simulink model "Turntable_sweep_2017"  (R2017b)
settings: Solver=ode4  StartTime=0.0  StopTime=10  FixedStep=0.0001  RelTol=1e-3
values from neighbouring files (symbols this model uses):
  b1 = 1 / taum    (= 1.01536120225)    [ESO.m]    (also in filter.m = 256.180350967; para_test.m)
  b2 = 1 / taue    (= 256.180350967)    [ESO.m]    (also in filter.m = 1.01536120225; para_test.m)
  beta1 = para.beta2    [ESO.m]    (also in filter.m = 221.733804685; myfun.m = x(6); para_test.m = 0.9528 * wq - b1 - b2)
  beta2 = para.beta3    [ESO.m]    (also in filter.m = 310055.997275; myfun.m = x(7); para_test.m = 1.4539 * wq * wq - b2 * beta1 - b1 * beta1 - b1 * b2)
  beta3 = para.beta4    [ESO.m]    (also in filter.m = 14508719.8625; myfun.m = x(8); para_test.m = 0.7426 * wq ^ 3 - b2 * beta2 - b1 * beta2 - b1 * b2 * beta1)
  beta4 = 0.2756 * wq ^ 4    (= 17593758835.7)    [filter.m]    (also in para_test.m = 0.2756 * wq ^ 4)
  fre = fre_array(i)    [sweep.m]
  gain = b0    (= 23249.4996924)    [para_test.m]
  J = 1.076    [sweep.m]
  Kps = 1.077250780790937e+02    (= 107.725078079)    [sweep.m]
  Kt = 24.812626200641272    (= 24.8126262006)    [sweep.m]
  Kv = 0.12    [sweep.m]
  L = 0.733240176511722    (= 0.733240176512)    [sweep.m]
  r = 80.116666666666666667    (= 80.1166666667)    [sweep.m]
  t_off = 10    [sweep.m]
  Type = 1    [sweep.m]
settings Model: Creator=Vera  LastModifiedBy=57531
settings SolverCC: AlgebraicLoopSolver=LineSearch
settings OptimizationCC: LifeSpan=inf
settings DebuggingCC: SFExecutionAtInitializationDiag=none
settings CodeAppCC: StateflowObjectComments=on

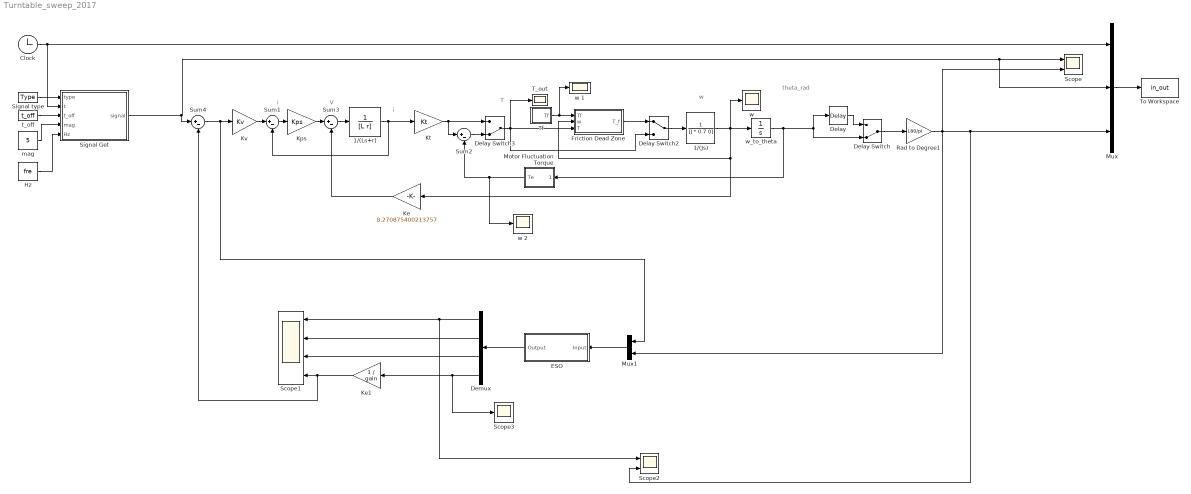
== system Turntable_sweep_2017 ==
  note: i
  note: w
  note: V
  note: i
  note: T
  note: theta_rad
  " Delay Switch" : ManualSwitch  CurrentSetting=0
  " Delay Switch2" : ManualSwitch
  " Delay Switch3" : ManualSwitch  CurrentSetting=0
  1/(Js) : TransferFcn  Denominator=[J * 0.7 0]
  1/(Ls+r) : TransferFcn  Denominator=[L r]
  Clock : Clock
  Delay : TransportDelay  DelayTime=0.003763900000000
  Demux : Demux
  ESO : Subsystem  mask{beta0=beta1, beta1=beta2, beta2=beta3, beta3=beta4, alpha1=0.5, alpha2=0.25, alpha3=0.125, delta1=0.01, delta2=0.01, delta3=0.01, h=0.0002, b0=gain}
  Friction Dead Zone : MATLAB Function  TreatAsAtomicUnit=on
  Hz : Constant  Value=fre
  Ke : Gain  Gain=8.270875400213757
  Ke1 : Gain  Gain=1 / gain
  Kps : Gain  Gain=Kps
  Kt : Gain  Gain=Kt
  Kv : Gain  Gain=Kv
  Motor Fluctuation Torque : Subsystem
  Mux : Mux  Inputs=3
  Mux1 : Mux  Inputs=2
  Rad to Degree1 : Gain  Gain=180/pi
  Scope : Scope  NumInputPorts=2
  Scope1 : Scope  NumInputPorts=4
  Scope2 : Scope  NumInputPorts=2
  Scope3 : Scope
  Signal Get : MATLAB Function  TreatAsAtomicUnit=on
  Signal type : Constant  Value=Type
  Sum{1..4} (4 alike) : Sum  Inputs=|+-
  T_out : Scope
  Tf : Subsystem
  To Workspace : ToWorkspace  VariableName=in_out  SampleTime=-1
  mag : Constant  Value=5
  t_off : Constant  Value=t_off
  "w " : Scope
  w 1 : Scope
  w 2 : Scope
  w_to_theta : Integrator
  wires:
  t_off/1 -> Signal Get/3(t_off)
  Clock/1 -> Mux/1, Signal Get/2(t)
  mag/1 -> Signal Get/4(mag)
  Hz/1 -> Signal Get/5(Hz)
  Kv/1 -> Sum1/1
  Motor Fluctuation Torque/1(Te) -> w 2/1, Sum2/2
  Tf/1(Tf) -> w 1/1, Friction Dead Zone/1(Tf)
  1/(Ls+r)/1 -> Sum1/2, Kt/1
  Sum3/1 -> 1/(Ls+r)/1
  Delay/1 -> " Delay Switch"/1
  w_to_theta/1 -> Delay/1, " Delay Switch"/2, Motor Fluctuation Torque/1(theta)
  " Delay Switch"/1 -> Rad to Degree1/1
  1/(Js)/1 -> "w "/1, w_to_theta/1, Friction Dead Zone/2(w), Ke/1
  " Delay Switch2"/1 -> 1/(Js)/1
  " Delay Switch3"/1 -> T_out/1, " Delay Switch2"/2, Friction Dead Zone/3(T)
  Ke/1 -> Sum3/2
  Sum2/1 -> " Delay Switch3"/2
  Sum1/1 -> Kps/1
  Kt/1 -> " Delay Switch3"/1, Sum2/1
  Kps/1 -> Sum3/1
  Mux/1 -> To Workspace/1
  Signal type/1 -> Signal Get/1(type)
  Rad to Degree1/1 -> Mux1/2, Scope2/2, Mux/3, Scope/2
  Demux/1 -> Scope2/1, Scope1/1
  Demux/2 -> Scope1/2
  Demux/3 -> Scope1/3
  Demux/4 -> Scope3/1, Ke1/1
  Friction Dead Zone/1(T_f) -> " Delay Switch2"/1
  Mux1/1 -> ESO/1(Input)
  ESO/1(Output) -> Demux/1
  Signal Get/1(signal) -> Sum4/1, Mux/2, Scope/1
  Ke1/1 -> Sum4/2, Scope1/4
  Sum4/1 -> Mux1/1, Kv/1

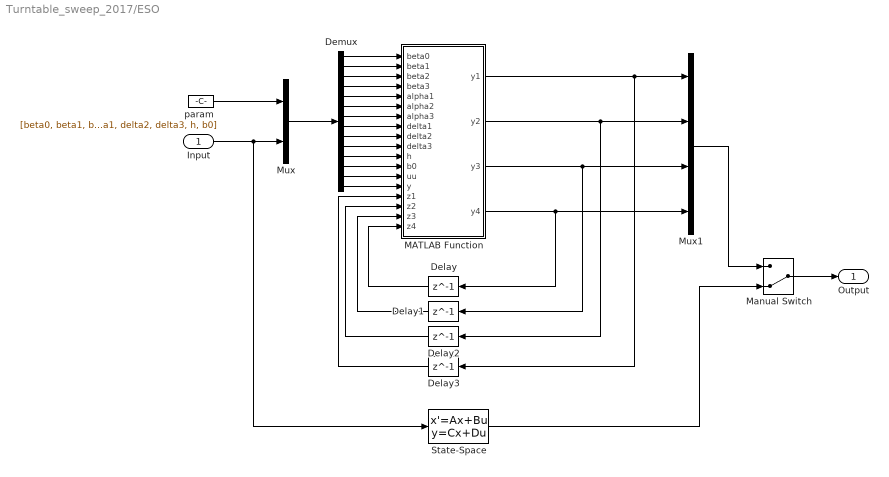
== system Turntable_sweep_2017/ESO ==
  Input : Inport
  Delay{,1..3} (4 alike) : Delay  DelayLength=1  InitialCondition=0
  Demux : Demux  Outputs=14
  MATLAB Function : MATLAB Function  TreatAsAtomicUnit=on
  Manual Switch : ManualSwitch  CurrentSetting=0
  Mux : Mux  Inputs=2
  Mux1 : Mux
  State-Space : StateSpace  A=[-beta0, 1, 0, 0; -beta1, 0, 1, 0; -beta2, -b1 * b2, -b1-b2, 1; -beta3, 0, 0, 0]  B=[0 beta0; 0 beta1; gain, beta2; 0, beta3]  C=diag([1 1 1 1])  D=[0 0; 0 0; 0 0; 0 0]  InitialCondition=0
  param : Constant  Value=[beta0, beta1, beta2, beta3, alpha1, alpha2, alpha3, delta1, delta2, delta3, h, b0]
  Output : Outport
  wires:
  Input/1 -> State-Space/1, Mux/2
  param/1 -> Mux/1
  Mux/1 -> Demux/1
  Demux/14 -> MATLAB Function/14(y)
  Demux/13 -> MATLAB Function/13(uu)
  Demux/12 -> MATLAB Function/12(b0)
  Demux/11 -> MATLAB Function/11(h)
  Demux/10 -> MATLAB Function/10(delta3)
  Demux/9 -> MATLAB Function/9(delta2)
  Demux/8 -> MATLAB Function/8(delta1)
  Demux/7 -> MATLAB Function/7(alpha3)
  Demux/6 -> MATLAB Function/6(alpha2)
  Demux/5 -> MATLAB Function/5(alpha1)
  Demux/4 -> MATLAB Function/4(beta3)
  Demux/3 -> MATLAB Function/3(beta2)
  Demux/2 -> MATLAB Function/2(beta1)
  Demux/1 -> MATLAB Function/1(beta0)
  Delay/1 -> MATLAB Function/18(z4)
  Delay1/1 -> MATLAB Function/17(z3)
  Delay2/1 -> MATLAB Function/16(z2)
  Delay3/1 -> MATLAB Function/15(z1)
  MATLAB Function/1(y1) -> Delay3/1, Mux1/1
  MATLAB Function/2(y2) -> Delay2/1, Mux1/2
  MATLAB Function/3(y3) -> Delay1/1, Mux1/3
  MATLAB Function/4(y4) -> Delay/1, Mux1/4
  State-Space/1 -> Manual Switch/2
  Mux1/1 -> Manual Switch/1
  Manual Switch/1 -> Output/1

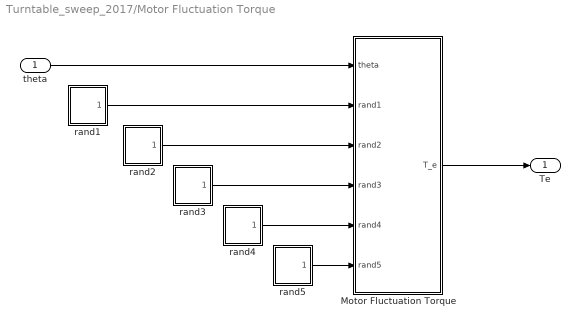
== system Turntable_sweep_2017/Motor Fluctuation Torque ==
  theta : Inport
  Motor Fluctuation Torque : MATLAB Function  TreatAsAtomicUnit=on
  rand1 : Subsystem
  rand2 : Subsystem
  rand3 : Subsystem
  rand4 : Subsystem
  rand5 : Subsystem
  Te : Outport
  wires:
  theta/1 -> Motor Fluctuation Torque/1(theta)
  rand1/1(rand1) -> Motor Fluctuation Torque/2(rand1)
  rand2/1(rand2) -> Motor Fluctuation Torque/3(rand2)
  rand3/1(rand3) -> Motor Fluctuation Torque/4(rand3)
  rand4/1(rand4) -> Motor Fluctuation Torque/5(rand4)
  rand5/1(rand5) -> Motor Fluctuation Torque/6(rand5)
  Motor Fluctuation Torque/1(T_e) -> Te/1

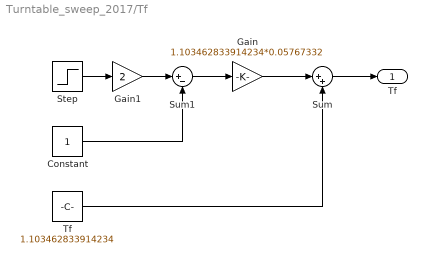
== system Turntable_sweep_2017/Tf ==
  Constant : Constant
  Gain : Gain  Gain=1.103462833914234*0.05767332
  Gain1 : Gain  Gain=2
  Step : Step  Time=0  After=rand  SampleTime=0
  Sum : Sum  Inputs=|++
  Sum1 : Sum  Inputs=|+-
  "Tf " : Constant  Value=1.103462833914234  VectorParams1D=off
  Tf : Outport
  wires:
  Gain/1 -> Sum/1
  "Tf "/1 -> Sum/2
  Sum/1 -> Tf/1
  Step/1 -> Gain1/1
  Gain1/1 -> Sum1/1
  Constant/1 -> Sum1/2
  Sum1/1 -> Gain/1

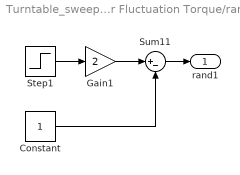
== system Turntable_sweep_2017/Motor Fluctuation Torque/rand1 ==
  Constant : Constant
  Gain1 : Gain  Gain=2
  Step1 : Step  Time=0  After=rand  SampleTime=0
  Sum11 : Sum  Inputs=|+-
  rand1 : Outport
  wires:
  Step1/1 -> Gain1/1
  Gain1/1 -> Sum11/1
  Constant/1 -> Sum11/2
  Sum11/1 -> rand1/1

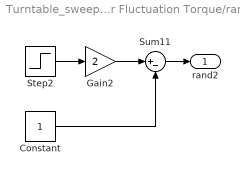
== system Turntable_sweep_2017/Motor Fluctuation Torque/rand2 ==
  Constant : Constant
  Gain2 : Gain  Gain=2
  Step2 : Step  Time=0  After=rand  SampleTime=0
  Sum11 : Sum  Inputs=|+-
  rand2 : Outport
  wires:
  Step2/1 -> Gain2/1
  Gain2/1 -> Sum11/1
  Constant/1 -> Sum11/2
  Sum11/1 -> rand2/1

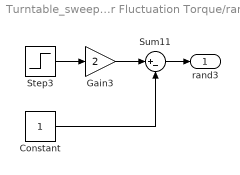
== system Turntable_sweep_2017/Motor Fluctuation Torque/rand3 ==
  Constant : Constant
  Gain3 : Gain  Gain=2
  Step3 : Step  Time=0  After=rand  SampleTime=0
  Sum11 : Sum  Inputs=|+-
  rand3 : Outport
  wires:
  Sum11/1 -> rand3/1
  Constant/1 -> Sum11/2
  Gain3/1 -> Sum11/1
  Step3/1 -> Gain3/1

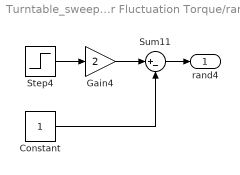
== system Turntable_sweep_2017/Motor Fluctuation Torque/rand4 ==
  Constant : Constant
  Gain4 : Gain  Gain=2
  Step4 : Step  Time=0  After=rand  SampleTime=0
  Sum11 : Sum  Inputs=|+-
  rand4 : Outport
  wires:
  Step4/1 -> Gain4/1
  Gain4/1 -> Sum11/1
  Constant/1 -> Sum11/2
  Sum11/1 -> rand4/1

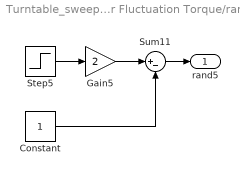
== system Turntable_sweep_2017/Motor Fluctuation Torque/rand5 ==
  Constant : Constant
  Gain5 : Gain  Gain=2
  Step5 : Step  Time=0  After=rand  SampleTime=0
  Sum11 : Sum  Inputs=|+-
  rand5 : Outport
  wires:
  Sum11/1 -> rand5/1
  Constant/1 -> Sum11/2
  Gain5/1 -> Sum11/1
  Step5/1 -> Gain5/1

== matlab function Turntable_sweep_2017/Signal Get ==
  data: type input; t input; t_off input; mag input; signal output; Hz input
function signal = fcn(type, t, t_off, mag, Hz)
signal = 0;
switch type
    case 1
        w = 2 * pi * Hz;
        if((t >= 0) && (t < 1))
            signal = t * mag * sin(w * t);
        elseif((t >= 1) && (t < t_off - 1))
            signal = mag * sin(w * t);
        elseif((t >= (t_off - 1)) && (t < t_off))
            signal = -mag * (t - t_off) * sin(w * t);
        else
            signal = 0;
        end
    case 2
        if t < 1
            signal = t * mag;
        elseif t >= 1 && t < (t_off - 1)
            signal = mag;
        elseif t >= (t_off - 1) && t < t_off
            signal = mag - (t_off - t) * mag;
        else
            signal = 0;
        end
        
end

== matlab function Turntable_sweep_2017/Friction Dead Zone ==
  data: Tf input; w input; T input; T_f output
function T_f = fcn(Tf,w,T)
if w==0
    if abs(T)<abs(Tf)
        T_f = 0;
    else
        T_f=sign(T)*(abs(T)-Tf);
    end
elseif w*T<0
    T_f=sign(T)*(abs(T)+Tf);
else 
        if abs(T)<abs(Tf)
            T_f = -sign(w)*(Tf-abs(T));
        else
            T_f=sign(T)*(abs(T)-Tf);
        end

end
end

== matlab function Turntable_sweep_2017/ESO/MATLAB Function ==
  data: beta0 input; y1 output; y2 output; y3 output; y4 output; beta1 input; beta2 input; beta3 input; alpha1 input; alpha2 input; alpha3 input; delta1 input; delta2 input; delta3 input; h input; b0 input; uu input; y input; z1 input; z2 input; z3 input; z4 input
function [y1, y2, y3, y4] = fcn(beta0,beta1, beta2, beta3, alpha1, alpha2, alpha3, delta1, delta2, delta3, h, b0, uu, y, z1, z2, z3, z4)
% 
% x0 = [z1, z2, z3, z4, beta0, beta1, beta2, beta3, alpha1, alpha2, alpha3, delta1, delta2, delta3, b0, uu, y];

dx = zeros(4, 1);
e = z1 - y;
dx(1) = z2 - beta0 * e;
dx(2) = z3 - beta1 * fal(e, 0.5, delta1);
dx(3) = z4 - beta2 * fal(e, 0.25, delta2) + b0 * uu - (1.015361202246130 + 2.561803509670808e+02) * z3 - (1.015361202246130 * 2.561803509670808e+02) * z2;
dx(4) = - beta3 * fal(e, 0.125, delta3);

% [~, tmpx] = ode23(@myfun, [0, h], x0); 
% [mm, ~] = size(tmpx);
% y1 = tmpx(mm, 1);
% y2 = tmpx(mm, 2);
% y3 = tmpx(mm, 3);
% y4 = tmpx(mm, 4);
y1 = z1 + h * dx(1);
y2 = z2 + h * dx(2);
y3 = z3 + h * dx(3);
y4 = z4 + h * dx(4);

== matlab function Turntable_sweep_2017/Motor Fluctuation Torque/Motor Fluctuation Torque ==
  data: T_e output; theta input; rand1 input; rand2 input; rand3 input; rand4 input; rand5 input
function T_e = fcn(theta,rand1,rand2,rand3,rand4,rand5)
T_p =0.432273269433135*(1+rand1*0.012015015613962)*cos(theta*7 +(48.13841636+0.050850865438431)*pi/180);
T_2p=0.035501355062786*(1+rand2*0.032198449030114)*cos(theta*14+(30.38979755+0.101746126073106)*pi/180);
T_4p=0.018930935537422*(1+rand3*0.028225982587057)*cos(theta*28+(285.7823597+0.203848223609672)*pi/180);
T_6p=0.012218243879728*(1+rand4*0.058230694793342)*cos(theta*42+(152.9148096+0.306666606518932)*pi/180);
T_45=0.009203318745614*(1+rand5*0.098213466988815)*cos(theta*45+(279.6898495+0.328827530537396)*pi/180);

T_e = (T_p + T_2p + T_4p + T_6p + T_45);
end
